simulink model "UKF"  (R2024a)
settings: Solver=VariableStepAuto  StartTime=0.0  StopTime=10.0  RelTol=1e-3
undefined symbols (not defined in the file): dt_imu, g_n, R_pos, R_vel, sigma_acc, sigma_ba, sigma_bg, sigma_gyr, ukf_alpha, ukf_beta, ukf_kappa
libraries: simulink x1
settings Model: DataDictionary=StateEstDict.sldd  Creator=89447  LastModifiedBy=89447

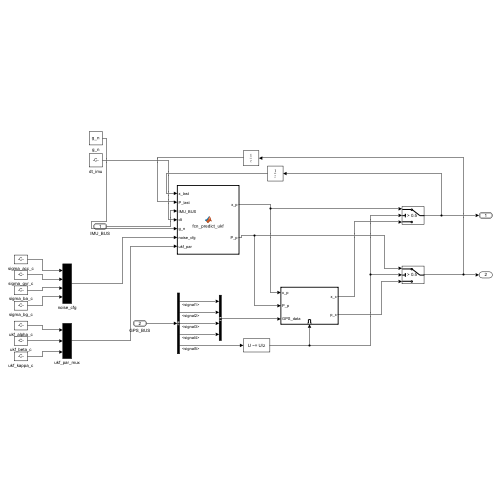
[thumbnail: Simulink's stored preview of the top-level diagram]
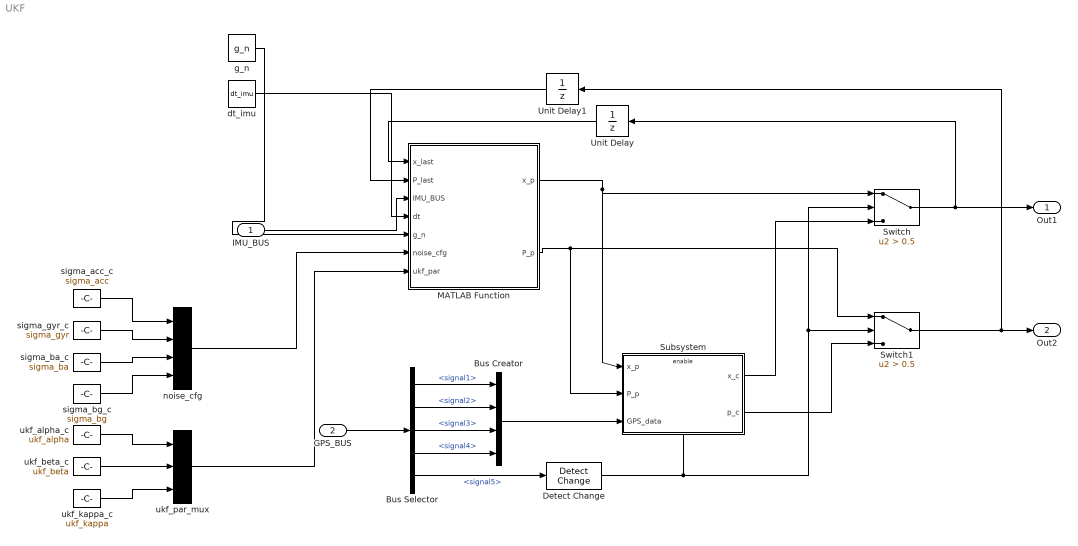
== system UKF ==
  IMU_BUS : Inport  OutDataTypeStr=Bus: IMU_BUS
  GPS_BUS : Inport  Port=2  OutDataTypeStr=Bus: GPS_BUS
  Bus Creator : BusCreator  Inputs=4
  Bus Selector : BusSelector  OutputSignals=signal1,signal2,signal3,signal4,signal5
  Detect Change : simulink/Logic and Bit Operations/Detect Change  vinit=0  OutDataTypeStr=boolean
  MATLAB Function : MATLAB Function  TreatAsAtomicUnit=on
  Subsystem : Subsystem
  Switch : Switch  Criteria=u2 > Threshold  Threshold=0.5  SaturateOnIntegerOverflow=off  InputSameDT=off
  Switch1 : Switch  Criteria=u2 > Threshold  Threshold=0.5  SaturateOnIntegerOverflow=off  InputSameDT=off
  Unit Delay : UnitDelay  SampleTime=-1  HasFrameUpgradeWarning=on
  Unit Delay1 : UnitDelay  SampleTime=-1  HasFrameUpgradeWarning=on
  dt_imu : Constant  Value=dt_imu  OutDataTypeStr=single
  g_n : Constant  Value=g_n  OutDataTypeStr=single
  noise_cfg : Mux
  sigma_acc_c : Constant  Value=sigma_acc  OutDataTypeStr=single
  sigma_ba_c : Constant  Value=sigma_ba  OutDataTypeStr=single
  sigma_bg_c : Constant  Value=sigma_bg  OutDataTypeStr=single
  sigma_gyr_c : Constant  Value=sigma_gyr  OutDataTypeStr=single
  ukf_alpha_c : Constant  Value=ukf_alpha  OutDataTypeStr=single
  ukf_beta_c : Constant  Value=ukf_beta  OutDataTypeStr=single
  ukf_kappa_c : Constant  Value=ukf_kappa  OutDataTypeStr=single
  ukf_par_mux : Mux  Inputs=3
  Out1 : Outport  OutDataTypeStr=Bus: StateEstBus
  Out2 : Outport  Port=2
  wires:
  MATLAB Function/1(x_p) -> Switch/1, Subsystem/1(x_p)
  Bus Selector/4 -> Bus Creator/4  "<signal4>"
  Bus Selector/3 -> Bus Creator/3  "<signal3>"
  IMU_BUS/1 -> MATLAB Function/3(IMU_BUS)
  Bus Selector/2 -> Bus Creator/2  "<signal2>"
  Bus Selector/1 -> Bus Creator/1  "<signal1>"
  Bus Creator/1 -> Subsystem/3(GPS_data)
  Detect Change/1 -> Subsystem/Enable, Switch/2, Switch1/2
  Bus Selector/5 -> Detect Change/1  "<signal5>"
  Unit Delay/1 -> MATLAB Function/1(x_last)
  MATLAB Function/2(P_p) -> Subsystem/2(P_p), Switch1/1
  Switch/1 -> Unit Delay/1, Out1/1
  Subsystem/1(x_c) -> Switch/3
  Unit Delay1/1 -> MATLAB Function/2(P_last)
  Subsystem/2(p_c) -> Switch1/3
  Switch1/1 -> Unit Delay1/1, Out2/1
  GPS_BUS/1 -> Bus Selector/1
  sigma_acc_c/1 -> noise_cfg/1
  sigma_gyr_c/1 -> noise_cfg/2
  sigma_ba_c/1 -> noise_cfg/3
  sigma_bg_c/1 -> noise_cfg/4
  g_n/1 -> MATLAB Function/5(g_n)
  dt_imu/1 -> MATLAB Function/4(dt)
  noise_cfg/1 -> MATLAB Function/6(noise_cfg)
  ukf_alpha_c/1 -> ukf_par_mux/1
  ukf_beta_c/1 -> ukf_par_mux/2
  ukf_kappa_c/1 -> ukf_par_mux/3
  ukf_par_mux/1 -> MATLAB Function/7(ukf_par)

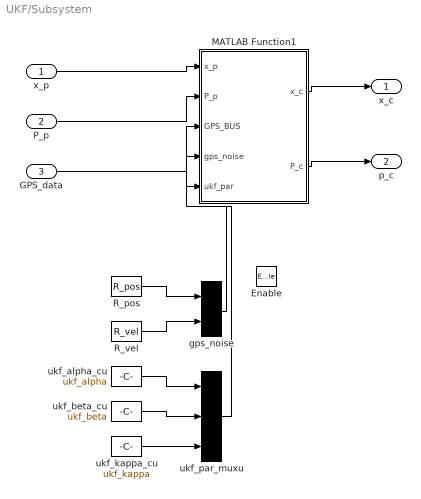
== system UKF/Subsystem ==
  x_p : Inport
  P_p : Inport  Port=2
  GPS_data : Inport  Port=3
  Enable : EnablePort
  MATLAB Function1 : MATLAB Function  TreatAsAtomicUnit=on
  R_pos : Constant  Value=R_pos  OutDataTypeStr=single
  R_vel : Constant  Value=R_vel  OutDataTypeStr=single
  gps_noise : Mux  Inputs=2
  ukf_alpha_cu : Constant  Value=ukf_alpha  OutDataTypeStr=single
  ukf_beta_cu : Constant  Value=ukf_beta  OutDataTypeStr=single
  ukf_kappa_cu : Constant  Value=ukf_kappa  OutDataTypeStr=single
  ukf_par_muxu : Mux  Inputs=3
  x_c : Outport
  p_c : Outport  Port=2
  wires:
  MATLAB Function1/1(x_c) -> x_c/1
  GPS_data/1 -> MATLAB Function1/3(GPS_BUS)
  x_p/1 -> MATLAB Function1/1(x_p)
  P_p/1 -> MATLAB Function1/2(P_p)
  MATLAB Function1/2(P_c) -> p_c/1
  R_pos/1 -> gps_noise/1
  R_vel/1 -> gps_noise/2
  gps_noise/1 -> MATLAB Function1/4(gps_noise)
  ukf_alpha_cu/1 -> ukf_par_muxu/1
  ukf_beta_cu/1 -> ukf_par_muxu/2
  ukf_kappa_cu/1 -> ukf_par_muxu/3
  ukf_par_muxu/1 -> MATLAB Function1/5(ukf_par)

== matlab function UKF/MATLAB Function ==
  data: x_last input; x_p output; P_last input; IMU_BUS input; P_p output; dt input; g_n input; noise_cfg input; ukf_par input
function [x_p, P_p] = fcn_predict_ukf(x_last, P_last, IMU_BUS, dt, g_n, noise_cfg, ukf_par)
% UKF 预测步 — Sigma 点传播
% Sigma 点生成在 15D 切空间上，注入流形后通过名义动力学传播
% ukf_par: [alpha; beta; kappa]

alpha = ukf_par(1); beta = ukf_par(2); kappa = ukf_par(3);
n = 15;
lambda = alpha^2 * (n + kappa) - n;

% --- 生成 Sigma 点 (切空间) ---
L = chol((n + lambda) * P_last, 'lower');
dX = zeros(n, 2*n+1);
for i = 1:n
    dX(:, i+1)   =  L(:, i);
    dX(:, n+i+1) = -L(:, i);
end

Wm = ones(2*n+1, 1) / (2*(n+lambda));
Wm(1) = lambda / (n+lambda);
Wc = Wm;
Wc(1) = Wc(1) + (1 - alpha^2 + beta);

% --- 将 Sigma 点映射到状态流形并传播 ---
X_p = zeros(16, 2*n+1);
for i = 1:2*n+1
    xi = x_last;
    if i > 1
        xi(1:3) = x_last(1:3) + dX(1:3, i);
        xi(4:6) = x_last(4:6) + dX(4:6, i);
        dqi = quat_exp(dX(7:9, i), 1.0);
        xi(7:10) = quat_mult(dqi, x_last(7:10));
        xi(7:10) = quat_normalize(xi(7:10));
        xi(11:13) = x_last(11:13) + dX(10:12, i);
        xi(14:16) = x_last(14:16) + dX(13:15, i);
    end
    X_p(:,i) = propagate_ukf(xi, IMU_BUS, dt, g_n);
end

% --- 重构名义状态 (四元数加权平均) ---
x_p = weighted_mean_ukf(X_p, Wm);

% --- 计算传播后各点在切空间中的偏离 ---
dX_p = zeros(n, 2*n+1);
for i = 1:2*n+1
    dX_p(1:3, i) = X_p(1:3, i) - x_p(1:3);
    dX_p(4:6, i) = X_p(4:6, i) - x_p(4:6);
    dq_err = quat_mult(X_p(7:10, i), [-x_p(7); x_p(8:10)]);
    dX_p(7:9, i) = 2 * dq_err(2:4);
    dX_p(10:12, i) = X_p(11:13, i) - x_p(11:13);
    dX_p(13:15, i) = X_p(14:16, i) - x_p(14:16);
end

% --- 加权协方差 ---
P_p = zeros(n, n);
for i = 1:2*n+1
    P_p = P_p + Wc(i) * (dX_p(:,i) * dX_p(:,i)');
end

% --- 添加过程噪声 ---
sigma_acc = noise_cfg(1); sigma_gyr = noise_cfg(2);
sigma_ba = noise_cfg(3); sigma_bg = noise_cfg(4);
Q_c = diag([sigma_acc*ones(1,3), sigma_gyr*ones(1,3), sigma_ba*ones(1,3), sigma_bg*ones(1,3)]);

accel_corr = IMU_BUS.Accel - x_last(11:13);
C_bn = quat2rotm(x_last(7:10));
G = zeros(15, 12);
G(4:6, 1:3) = -C_bn; G(7:9, 4:6) = -eye(3);
G(10:12, 7:9) = eye(3); G(13:15, 10:12) = eye(3);
Q_d = G * Q_c * G' * dt;

P_p = P_p + Q_d;
P_p = (P_p + P_p') / 2;
end

function x_new = propagate_ukf(x, IMU_BUS, dt, g_n)
    p = x(1:3); v = x(4:6); q = x(7:10);
    ba = x(11:13); bg = x(14:16);
    accel_corr = IMU_BUS.Accel - ba;
    omega_corr = IMU_BUS.Gyro - bg;
    dq = quat_exp(omega_corr, dt);
    q_p = quat_mult(q, dq);
    q_p = quat_normalize(q_p);
    C_bn = quat2rotm(q);
    a_n = C_bn * accel_corr + g_n;
    v_p = v + a_n * dt;
    p_p = p + v * dt + 0.5 * a_n * dt^2;
    x_new = [p_p; v_p; q_p; ba; bg];
end

function x_mean = weighted_mean_ukf(X, W)
    x_mean = zeros(16, 1);
    x_mean(1:3) = X(1:3,:) * W;
    x_mean(4:6) = X(4:6,:) * W;
    M = zeros(4, 4);
    for j = 1:size(X,2)
        qj = X(7:10, j);
        M = M + W(j) * (qj * qj');
    end
    [V, D] = eig(M);
    [~, idx] = max(diag(real(D)));
    q_mean = real(V(:, idx));
    if q_mean(1) < 0, q_mean = -q_mean; end
    x_mean(7:10) = q_mean / norm(q_mean);
    x_mean(11:13) = X(11:13,:) * W;
    x_mean(14:16) = X(14:16,:) * W;
end

== matlab function UKF/Subsystem/MATLAB Function1 ==
  data: x_p input; x_c output; P_p input; GPS_BUS input; P_c output; gps_noise input; ukf_par input
function [x_c, P_c] = fcn_update_ukf(x_p, P_p, GPS_BUS, gps_noise, ukf_par)
% UKF 更新步 — Sigma 点通过观测模型传播
% 在切空间生成 Sigma 点，注入流形后计算观测统计量与互协方差

alpha = ukf_par(1); beta = ukf_par(2); kappa = ukf_par(3);
n = 15;
lambda = alpha^2 * (n + kappa) - n;

% --- 生成 Sigma 点 (切空间) ---
L = chol((n + lambda) * P_p, 'lower');
dX = zeros(n, 2*n+1);
for i = 1:n
    dX(:, i+1)   =  L(:, i);
    dX(:, n+i+1) = -L(:, i);
end

Wm = ones(2*n+1, 1) / (2*(n+lambda));
Wm(1) = lambda / (n+lambda);
Wc = Wm;
Wc(1) = Wc(1) + (1 - alpha^2 + beta);

% --- 将 Sigma 点映射到状态流形，通过观测函数 ---
Z = zeros(6, 2*n+1);
for i = 1:2*n+1
    xi = x_p;
    if i > 1
        xi(1:3) = x_p(1:3) + dX(1:3, i);
        xi(4:6) = x_p(4:6) + dX(4:6, i);
        dqi = quat_exp(dX(7:9, i), 1.0);
        xi(7:10) = quat_mult(dqi, x_p(7:10));
        xi(7:10) = quat_normalize(xi(7:10));
        xi(11:13) = x_p(11:13) + dX(10:12, i);
        xi(14:16) = x_p(14:16) + dX(13:15, i);
    end
    Z(:,i) = [xi(1:3); xi(4:6)];
end

% --- 观测统计量 ---
z_mean = Z * Wm;

R_pos = gps_noise(1); R_vel = gps_noise(2);
R = diag([R_pos*ones(1,3), R_vel*ones(1,3)]);

P_zz = R;
P_xz = zeros(n, 6);
for i = 1:2*n+1
    dz = Z(:,i) - z_mean;
    P_zz = P_zz + Wc(i) * (dz * dz');
    P_xz = P_xz + Wc(i) * (dX(:,i) * dz');
end

% --- 卡尔曼增益与状态修正 ---
z = [GPS_BUS.Lat; GPS_BUS.Lon; GPS_BUS.Alt; GPS_BUS.Velocity];
K = P_xz / P_zz;
delta_x = K * (z - z_mean);

% --- 修正量合入全状态 (流形 retraction) ---
x_c = x_p;
x_c(1:3) = x_p(1:3) + delta_x(1:3);
x_c(4:6) = x_p(4:6) + delta_x(4:6);
dq = quat_exp(delta_x(7:9), 1.0);
x_c(7:10) = quat_mult(dq, x_p(7:10));
x_c(7:10) = quat_normalize(x_c(7:10));
x_c(11:13) = x_p(11:13) + delta_x(10:12);
x_c(14:16) = x_p(14:16) + delta_x(13:15);

% --- 协方差更新 ---
P_c = P_p - K * P_zz * K';
P_c = (P_c + P_c') / 2;
end
